simulink model "simple_unctrlld_mdl"  (Simulink 8.2)
settings: Solver=ode45  StartTime=0.0  StopTime=.06  RelTol=1e-3
libraries: powerlib x22
settings Model: Creator=Pratp_000  LastModifiedBy=Pratp_000
settings DataIOCC: SignalLoggingSaveFormat=Dataset
settings OptimizationCC: ExpressionDepthLimit=128
settings DebuggingCC: FcnCallInpInsideContextMsg=EnableAllAsError  StateNameClashWarn=none
settings GRTTargetCC: CombineOutputUpdateFcns=on  GRTInterface=off

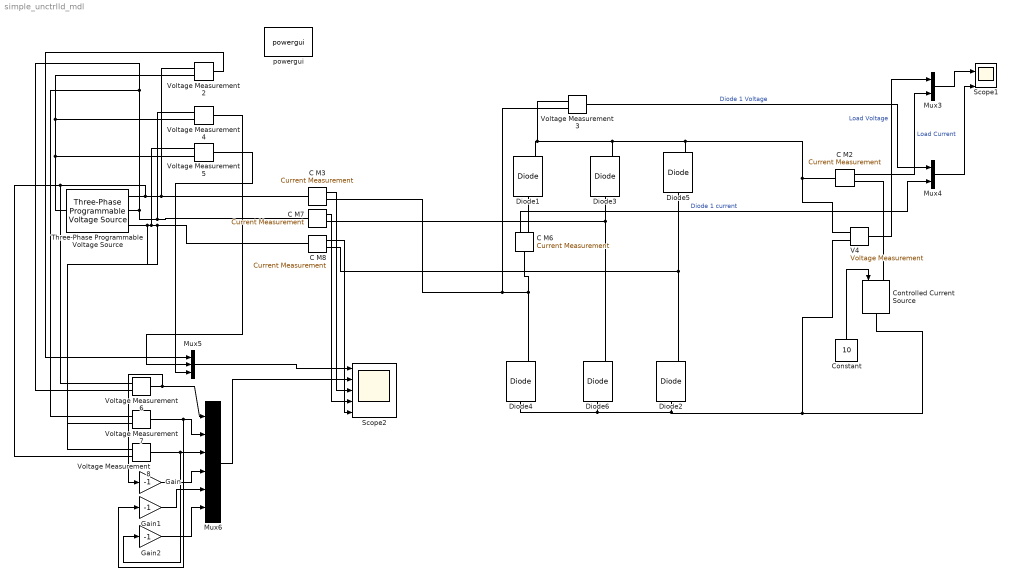
== system simple_unctrlld_mdl ==
  C M{2..3,6..8} (5 alike) : powerlib/Measurements/Current Measurement  PhasorSimulation=off  OutputType=Complex  PSBequivalent=0
  Constant : Constant  Value=10
  Controlled Current Source : powerlib/Electrical Sources/Controlled Current Source  Initialize=on  Source_Type=DC  Amplitude=10  Phase=0  Frequency=0  Measurements=None
  Diode{1..6} (6 alike) : powerlib/Power Electronics/Diode  Ron=0.001  Lon=0  Vf=0.8  IC=0  UseSnubber=off  Rs=500  Cs=250e-9  Measurements=on
  Gain : Gain  Gain=-1
  Gain1 : Gain  Gain=-1
  Gain2 : Gain  Gain=-1
  Mux3 : Mux  Inputs=2
  Mux4 : Mux  Inputs=2
  Mux5 : Mux  Inputs=3
  Mux6 : Mux  Inputs=6
  Scope1 : Scope  NumInputPorts=4
      settings: ShowLegends=on  YMin=0~-5~-5~-5  YMax=50~5~5~5  Decimation=3
  Scope2 : Scope  NumInputPorts=5
      settings: YMin=-200~-350~-0.459708~-2.18199~2.39011  YMax=200~200~-0.415926~-1.97419~2.64171  SaveName=pp  Decimation=3
  Three-Phase Programmable Voltage Source : powerlib/Electrical Sources/Three-Phase Programmable Voltage Source  PositiveSequence="[220  0 50]"  VariationEntity=None  VariationType=Table of time-amplitude pairs  VariationTypeAlt=Step  VariationStep=0.5  VariationRate=10  VariationMagnitude=0.3  VariationFrequency=2  VariationTiming=[1 2]  VariationPhaseA=off  Amplitudes=[1 0.8 1.2 1.0]  TimeValues=[0 0.1 0.15 0.2]  HarmonicGeneration=off  HarmonicA=[3 0.2 -25 0]  HarmonicB=[2 0.15 35 2]  Timing="[0.05  3]"  BusType=swing  Pref=0  Qref=0  Qmin=-inf  Qmax=inf
  V4 : powerlib/Measurements/Voltage Measurement  PhasorSimulation=off  OutputType=Complex  PSBequivalent=0
  Voltage Measurement{2..8} (7 alike) : powerlib/Measurements/Voltage Measurement  PhasorSimulation=off  OutputType=Complex  PSBequivalent=0
  powergui : powerlib/powergui  Priority=1  SimulationMode=Discrete  SolverType=Tustin  SampleTime=10e-6  frequency=60  SPID=off  DisableSnubberDevices=off  DisableRonSwitches=off  DisableVfSwitches=off  SwTol=0  Interpol=off  DisplayEquations=off  frequencyindice=50  Pbase=100e6  ErrMax=1e-4  Iterations=50  UnitsV=kV  UnitsW=MW  FunctionMessages=off  echomessages=off  HookPort=off  EnableUseOfTLC=off  x0status=blocks  RestoreLinks=warning  ResistiveCurrentMeasurement=off  Frange=[0:2:500]  Ylog=off  Xlog=on  ShowGrid=off  save=off  variable=ZData  structure=ScopeData1  ZoomFFT=on  StartTime=0.1  cycles=1  DisplayStyle=1  fundamental=50  FreqAxis=on  MaxFrequency=1000  frequencyindicesteady=1  RmsSteady=1  display=off  Ts=0  methode=off
  wires:
  Voltage Measurement2/1 -> Mux5/1
  C M3/1 -> Scope2/3
  C M2/1 -> Mux3/2  "Load Current"
  V4/1 -> Mux3/1  "Load Voltage"
  Mux3/1 -> Scope1/2
  Voltage Measurement3/1 -> Mux4/1  "Diode 1 Voltage"
  Mux4/1 -> Scope1/4
  C M6/1 -> Mux4/2  "Diode 1 current"
  Voltage Measurement4/1 -> Mux5/2
  Voltage Measurement5/1 -> Mux5/3
  Mux5/1 -> Scope2/1
  Voltage Measurement6/1 -> Gain/1, Mux6/1
  Voltage Measurement7/1 -> Gain1/1, Mux6/2
  Voltage Measurement8/1 -> Gain2/1, Mux6/3
  Mux6/1 -> Scope2/2
  C M7/1 -> Scope2/4
  C M8/1 -> Scope2/5
  Gain/1 -> Mux6/4
  Gain1/1 -> Mux6/5
  Gain2/1 -> Mux6/6
  Constant/1 -> Controlled Current Source/1
  connections:
  Diode3/LConn1 -- C M7/RConn1 -- Diode6/RConn1
  Diode5/LConn1 -- C M8/RConn1 -- Diode2/RConn1
  Diode4/LConn1 -- Diode6/LConn1 -- Controlled Current Source/RConn1 -- V4/LConn2 -- Diode2/LConn1
  C M2/RConn1 -- Controlled Current Source/LConn1
  Voltage Measurement2/LConn2 -- Three-Phase Programmable Voltage Source/LConn1 -- Voltage Measurement5/LConn2 -- Voltage Measurement4/LConn2
  Voltage Measurement2/LConn1 -- C M3/LConn1 -- Voltage Measurement8/LConn2 -- Voltage Measurement6/LConn1 -- Three-Phase Programmable Voltage Source/RConn1
  Diode1/LConn1 -- C M6/RConn1
  C M6/LConn1 -- C M3/RConn1 -- Voltage Measurement3/LConn2 -- Diode4/RConn1
  C M7/LConn1 -- Voltage Measurement4/LConn1 -- Voltage Measurement7/LConn1 -- Voltage Measurement6/LConn2 -- Three-Phase Programmable Voltage Source/RConn2
  C M8/LConn1 -- Voltage Measurement8/LConn1 -- Three-Phase Programmable Voltage Source/RConn3 -- Voltage Measurement7/LConn2 -- Voltage Measurement5/LConn1
  V4/LConn1 -- Diode1/RConn1 -- Voltage Measurement3/LConn1 -- Diode3/RConn1 -- Diode5/RConn1 -- C M2/LConn1
